simulink model "Sim_AdaptiveFinalazo_ultimo_adaptativo"  (Simulink 7.9)
settings: Solver=ode45  SolverMode=SingleTasking  StartTime=0.0  StopTime=10.0  RelTol=1e-3
values from neighbouring files (symbols this model uses):
  B = [0;1]    [leyDeControl.m]
  gamma = 0.01 *eye(2)    [leyDeControl.m]
  In = 0.002381    [parametros_ultimo.m]
  Kd = 10000    [leyDeControl.m]    (also in parametros_ultimo.m)
  Kn = 0.0347    [parametros_ultimo.m]
  Kp = 100000    [leyDeControl.m]    (also in parametros_ultimo.m)
  Ln = 0.2175    [parametros_ultimo.m]
  Mn = 0.1047708    [parametros_ultimo.m]
  P = lyap(A,Q)    [leyDeControl.m]    (also in parametros_ultimo.m = lyap(a,0.2*eye(2)))
undefined symbols (not defined in the file or in its folder): Kfn
libraries: simulink x4
settings Model: Creator=Harryth  LastModifiedBy=i95sa
settings DataIOCC: SignalLoggingSaveFormat=Dataset
settings OptimizationCC: BlockReduction=off  BooleanDataType=off  ExpressionDepthLimit=128
settings DebuggingCC: SaveWithParameterizedLinksMsg=none  SignalResolutionControl=TryResolveAllWithWarning  SolverPrmCheckMsg=none  FrameProcessingCompatibilityMsg=error  StateNameClashWarn=none
settings HardwareCC: TargetUnknown=on
settings CodeAppCC: CustomSymbolStrType=$N$R$M_T
settings GRTTargetCC: CodeReplacementLibrary=C89/C90 (ANSI)

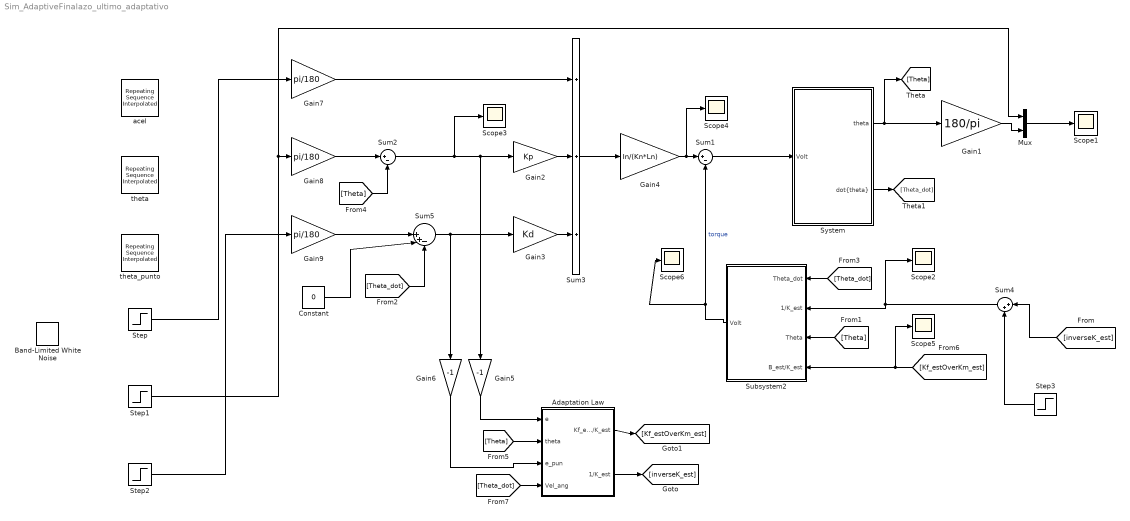
== system Sim_AdaptiveFinalazo_ultimo_adaptativo ==
  Adaptation Law : Subsystem
  Band-Limited White Noise : simulink/Sources/Band-Limited White Noise  Cov=[0.00001]  Ts=0.1  seed=[23341]
  Constant : Constant  Value=0
  Gain1 : Gain  Gain=180/pi
  Gain2 : Gain  Gain=Kp
  Gain3 : Gain  Gain=Kd
  Gain4 : Gain  Gain=In/(Kn*Ln)
  Gain5 : Gain  Gain=-1
  Gain6 : Gain  Gain=-1
  Gain7 : Gain  Gain=pi/180
  Gain8 : Gain  Gain=pi/180
  Gain9 : Gain  Gain=pi/180
  Mux : Mux  Inputs=2
  Scope{1..6} (6 alike) : Scope
      Scope1 settings: TimeRange=auto  MaxDataPoints=5000  SaveName=x1  YMin=-41.89754  YMax=4.65528  SampleTime=-1  DataFormat=Array
      Scope2 settings: TimeRange=auto  MaxDataPoints=5000  SaveName=x  YMin=35.99194  YMax=36.21018  SampleTime=-1  DataFormat=Array
      Scope3 settings: TimeRange=auto  LimitDataPoints=on  MaxDataPoints=5000  SaveToWorkspace=off  SaveName=ScopeData  YMin=-10  YMax=10  SampleTime=-1  DataFormat=Array
      Scope4 settings: TimeRange=auto  LimitDataPoints=on  MaxDataPoints=5000  SaveToWorkspace=off  SaveName=ScopeData  YMin=-4609.88714  YMax=40404.40736  SampleTime=-1  DataFormat=Array
      Scope5 settings: TimeRange=auto  MaxDataPoints=5000  SaveName=x2  YMin=-0.88055  YMax=0.67421  SampleTime=-1  DataFormat=Array
      Scope6 settings: TimeRange=auto  LimitDataPoints=on  MaxDataPoints=5000  SaveToWorkspace=off  SaveName=ScopeData  YMin=-6.67771  YMax=27.31814  SampleTime=-1  DataFormat=Array
  Step : Step  Time=0  After=0  SampleTime=0
  Step1 : Step  Time=0  After=0  SampleTime=0
  Step2 : Step  Time=0  After=0  SampleTime=0
  Step3 : Step  Time=5  After=pi/18  SampleTime=0
  Subsystem2 : Subsystem
  Sum1 : Sum  Inputs=|+-
  Sum2 : Sum  Inputs=|+-
  Sum3 : Sum  Inputs=+++
  Sum4 : Sum  Inputs=|++
  Sum5 : Sum  Inputs=||++-
  System : Subsystem
  acel : simulink/Sources/Repeating Sequence Interpolated  OutValues=|  TimeValues=|  LookUpMeth=Interpolation-Use End Values  tsamp=0.01  OutMin=[]  OutMax=[]  OutDataTypeStr=double  OutputDataTypeScalingMode=double  OutDataType=fixdt(0,8)  OutScaling=2^-10
      OutValues=|
      | [3.12
      | 3.06
      | 3.00
      | 2.93
      | 2.87
      | 2.81
      | 2.75
      | 2.68
      | 2.62
      | 2.56
      | 2.50
      | 2.43
      | 2.37
      | 2.31
      | 2.25
      | 2.18
      | 2.12
      | 2.06
      | 2.00
      | 1.93
      | 1.87
      | 1.81
      | 1.75
      | 1.68
      | 1.62
      | 1.56
      | 1.50
      | 1.44
      | 1.37
      | 1.31
      | 1.25
      | 1.19
      | 1.12
      | 1.06
      | 1.00
      | 0.94
      | 0.87
      | 0.81
      | 0.75
      | 0.69
      | 0.62
      | 0.56
      | 0.50
      | 0.44
      | 0.37
      | 0.31
      | 0.25
      | 0.19
      | 0.12
      | 0.06
      | 0.00
      | -0.06
      | -0.12
      | -0.19
      | -0.25
      | -0.31
      | -0.37
      | -0.44
      | -0.50
      | -0.56
      | -0.62
      | -0.69
      | -0.75
      | -0.81
      | -0.87
      | -0.94
      | -1.00
      | -1.06
      | -1.12
      | -1.19
      | -1.25
      | -1.31
      | -1.37
      | -1.44
      | -1.50
      | -1.56
      | -1.62
      | -1.68
      | -1.75
      | -1.81
      | -1.87
      | -1.93
      | -2.00
      | -2.06
      | -2.12
      | -2.18
      | -2.25
      | -2.31
      | -2.37
      | -2.43
      | -2.50
      | -2.56
      | -2.62
      | -2.68
      | -2.75
      | -2.81
      | -2.87
      | -2.93
      | -3.00
      | -3.06
      | -3.12
      | ].'
      TimeValues=|
      | [0.00
      | 0.10
      | 0.20
      | 0.30
      | 0.40
      | 0.50
      | 0.60
      | 0.70
      | 0.80
      | 0.90
      | 1.00
      | 1.10
      | 1.20
      | 1.30
      | 1.40
      | 1.50
      | 1.60
      | 1.70
      | 1.80
      | 1.90
      | 2.00
      | 2.10
      | 2.20
      | 2.30
      | 2.40
      | 2.50
      | 2.60
      | 2.70
      | 2.80
      | 2.90
      | 3.00
      | 3.10
      | 3.20
      | 3.30
      | 3.40
      | 3.50
      | 3.60
      | 3.70
      | 3.80
      | 3.90
      | 4.00
      | 4.10
      | 4.20
      | 4.30
      | 4.40
      | 4.50
      | 4.60
      | 4.70
      | 4.80
      | 4.90
      | 5.00
      | 5.10
      | 5.20
      | 5.30
      | 5.40
      | 5.50
      | 5.60
      | 5.70
      | 5.80
      | 5.90
      | 6.00
      | 6.10
      | 6.20
      | 6.30
      | 6.40
      | 6.50
      | 6.60
      | 6.70
      | 6.80
      | 6.90
      | 7.00
      | 7.10
      | 7.20
      | 7.30
      | 7.40
      | 7.50
      | 7.60
      | 7.70
      | 7.80
      | 7.90
      | 8.00
      | 8.10
      | 8.20
      | 8.30
      | 8.40
      | 8.50
      | 8.60
      | 8.70
      | 8.80
      | 8.90
      | 9.00
      | 9.10
      | 9.20
      | 9.30
      | 9.40
      | 9.50
      | 9.60
      | 9.70
      | 9.80
      | 9.90
      | 10.00].'
  theta : simulink/Sources/Repeating Sequence Interpolated  OutValues=|  TimeValues=|  LookUpMeth=Interpolation-Use End Values  tsamp=0.01  OutMin=[]  OutMax=[]  OutDataTypeStr=double  OutputDataTypeScalingMode=double  OutDataType=fixdt(0,8)  OutScaling=2^-10
      OutValues=|
      | [-37.00
      | -36.98
      | -36.94
      | -36.86
      | -36.76
      | -36.62
      | -36.46
      | -36.27
      | -36.05
      | -35.81
      | -35.54
      | -35.25
      | -34.93
      | -34.59
      | -34.23
      | -33.84
      | -33.43
      | -33.00
      | -32.55
      | -32.08
      | -31.59
      | -31.08
      | -30.56
      | -30.01
      | -29.45
      | -28.88
      | -28.28
      | -27.67
      | -27.05
      | -26.42
      | -25.77
      | -25.11
      | -24.43
      | -23.75
      | -23.05
      | -22.35
      | -21.63
      | -20.91
      | -20.18
      | -19.44
      | -18.70
      | -17.94
      | -17.19
      | -16.42
      | -15.66
      | -14.89
      | -14.11
      | -13.34
      | -12.56
      | -11.78
      | -11.00
      | -10.22
      | -9.44
      | -8.66
      | -7.89
      | -7.11
      | -6.34
      | -5.58
      | -4.81
      | -4.06
      | -3.30
      | -2.56
      | -1.82
      | -1.09
      | -0.37
      | 0.35
      | 1.05
      | 1.75
      | 2.43
      | 3.11
      | 3.77
      | 4.42
      | 5.05
      | 5.67
      | 6.28
      | 6.88
      | 7.45
      | 8.01
      | 8.56
      | 9.08
      | 9.59
      | 10.08
      | 10.55
      | 11.00
      | 11.43
      | 11.84
      | 12.23
      | 12.59
      | 12.93
      | 13.25
      | 13.54
      | 13.81
      | 14.05
      | 14.27
      | 14.46
      | 14.62
      | 14.76
      | 14.86
      | 14.94
      | 14.98
      | 15.00
      | ].'
      TimeValues=|
      | [0.00
      | 0.10
      | 0.20
      | 0.30
      | 0.40
      | 0.50
      | 0.60
      | 0.70
      | 0.80
      | 0.90
      | 1.00
      | 1.10
      | 1.20
      | 1.30
      | 1.40
      | 1.50
      | 1.60
      | 1.70
      | 1.80
      | 1.90
      | 2.00
      | 2.10
      | 2.20
      | 2.30
      | 2.40
      | 2.50
      | 2.60
      | 2.70
      | 2.80
      | 2.90
      | 3.00
      | 3.10
      | 3.20
      | 3.30
      | 3.40
      | 3.50
      | 3.60
      | 3.70
      | 3.80
      | 3.90
      | 4.00
      | 4.10
      | 4.20
      | 4.30
      | 4.40
      | 4.50
      | 4.60
      | 4.70
      | 4.80
      | 4.90
      | 5.00
      | 5.10
      | 5.20
      | 5.30
      | 5.40
      | 5.50
      | 5.60
      | 5.70
      | 5.80
      | 5.90
      | 6.00
      | 6.10
      | 6.20
      | 6.30
      | 6.40
      | 6.50
      | 6.60
      | 6.70
      | 6.80
      | 6.90
      | 7.00
      | 7.10
      | 7.20
      | 7.30
      | 7.40
      | 7.50
      | 7.60
      | 7.70
      | 7.80
      | 7.90
      | 8.00
      | 8.10
      | 8.20
      | 8.30
      | 8.40
      | 8.50
      | 8.60
      | 8.70
      | 8.80
      | 8.90
      | 9.00
      | 9.10
      | 9.20
      | 9.30
      | 9.40
      | 9.50
      | 9.60
      | 9.70
      | 9.80
      | 9.90
      | 10.00].'
  theta_punto : simulink/Sources/Repeating Sequence Interpolated  OutValues=|  TimeValues=|  LookUpMeth=Interpolation-Use End Values  tsamp=0.01  OutMin=[]  OutMax=[]  OutDataTypeStr=double  OutputDataTypeScalingMode=double  OutDataType=fixdt(0,8)  OutScaling=2^-10
      OutValues=|
      | [0.00
      | 0.31
      | 0.61
      | 0.91
      | 1.20
      | 1.48
      | 1.76
      | 2.03
      | 2.30
      | 2.56
      | 2.81
      | 3.05
      | 3.29
      | 3.53
      | 3.76
      | 3.98
      | 4.19
      | 4.40
      | 4.61
      | 4.80
      | 4.99
      | 5.18
      | 5.35
      | 5.53
      | 5.69
      | 5.85
      | 6.00
      | 6.15
      | 6.29
      | 6.42
      | 6.55
      | 6.67
      | 6.79
      | 6.90
      | 7.00
      | 7.10
      | 7.19
      | 7.27
      | 7.35
      | 7.42
      | 7.49
      | 7.55
      | 7.60
      | 7.65
      | 7.69
      | 7.72
      | 7.75
      | 7.77
      | 7.79
      | 7.80
      | 7.80
      | 7.80
      | 7.79
      | 7.77
      | 7.75
      | 7.72
      | 7.69
      | 7.65
      | 7.60
      | 7.55
      | 7.49
      | 7.42
      | 7.35
      | 7.27
      | 7.19
      | 7.10
      | 7.00
      | 6.90
      | 6.79
      | 6.67
      | 6.55
      | 6.42
      | 6.29
      | 6.15
      | 6.00
      | 5.85
      | 5.69
      | 5.53
      | 5.35
      | 5.18
      | 4.99
      | 4.80
      | 4.61
      | 4.40
      | 4.19
      | 3.98
      | 3.76
      | 3.53
      | 3.29
      | 3.05
      | 2.81
      | 2.56
      | 2.30
      | 2.03
      | 1.76
      | 1.48
      | 1.20
      | 0.91
      | 0.61
      | 0.31
      | 0.00
      | ].'
      TimeValues=|
      | [0.00
      | 0.10
      | 0.20
      | 0.30
      | 0.40
      | 0.50
      | 0.60
      | 0.70
      | 0.80
      | 0.90
      | 1.00
      | 1.10
      | 1.20
      | 1.30
      | 1.40
      | 1.50
      | 1.60
      | 1.70
      | 1.80
      | 1.90
      | 2.00
      | 2.10
      | 2.20
      | 2.30
      | 2.40
      | 2.50
      | 2.60
      | 2.70
      | 2.80
      | 2.90
      | 3.00
      | 3.10
      | 3.20
      | 3.30
      | 3.40
      | 3.50
      | 3.60
      | 3.70
      | 3.80
      | 3.90
      | 4.00
      | 4.10
      | 4.20
      | 4.30
      | 4.40
      | 4.50
      | 4.60
      | 4.70
      | 4.80
      | 4.90
      | 5.00
      | 5.10
      | 5.20
      | 5.30
      | 5.40
      | 5.50
      | 5.60
      | 5.70
      | 5.80
      | 5.90
      | 6.00
      | 6.10
      | 6.20
      | 6.30
      | 6.40
      | 6.50
      | 6.60
      | 6.70
      | 6.80
      | 6.90
      | 7.00
      | 7.10
      | 7.20
      | 7.30
      | 7.40
      | 7.50
      | 7.60
      | 7.70
      | 7.80
      | 7.90
      | 8.00
      | 8.10
      | 8.20
      | 8.30
      | 8.40
      | 8.50
      | 8.60
      | 8.70
      | 8.80
      | 8.90
      | 9.00
      | 9.10
      | 9.20
      | 9.30
      | 9.40
      | 9.50
      | 9.60
      | 9.70
      | 9.80
      | 9.90
      | 10.00].'
  wires:
  System/2("dot{theta}") -> [Theta_dot]
  Sum1/1 -> System/1(Volt)
  Subsystem2/1(Volt) -> Scope6/1, Sum1/2  "torque"
  Sum3/1 -> Gain4/1
  Step/1 -> Gain7/1
  Sum4/1 -> Scope2/1, Subsystem2/2(1/K_est)
  [Theta] -> Subsystem2/3(Theta)
  [Theta_dot] -> Subsystem2/1(Theta_dot)
  [Kf_estOverKm_est] -> Scope5/1, Subsystem2/4(B_est/K_est)
  System/1(theta) -> Gain1/1, [Theta]
  [Theta] -> Sum2/2
  [Theta_dot] -> Sum5/3
  Gain2/1 -> Sum3/2
  Gain3/1 -> Sum3/3
  Gain4/1 -> Scope4/1, Sum1/1
  Step1/1 -> Mux/1, Gain8/1
  Step2/1 -> Gain9/1
  Sum5/1 -> Gain3/1, Gain6/1
  [Theta] -> Adaptation Law/2(theta)
  Sum2/1 -> Gain2/1, Gain5/1, Scope3/1
  [Theta_dot] -> Adaptation Law/4("Vel_ang ")
  Gain5/1 -> Adaptation Law/1(e)
  Gain6/1 -> Adaptation Law/3("e_pun ")
  Adaptation Law/1(Kf_est/K_est) -> [Kf_estOverKm_est]
  Adaptation Law/2(1/K_est) -> [inverseK_est]
  Gain7/1 -> Sum3/1
  Gain8/1 -> Sum2/1
  Gain9/1 -> Sum5/1
  Mux/1 -> Scope1/1
  Gain1/1 -> Mux/2
  Constant/1 -> Sum5/2
  [inverseK_est] -> Sum4/1
  Step3/1 -> Sum4/2

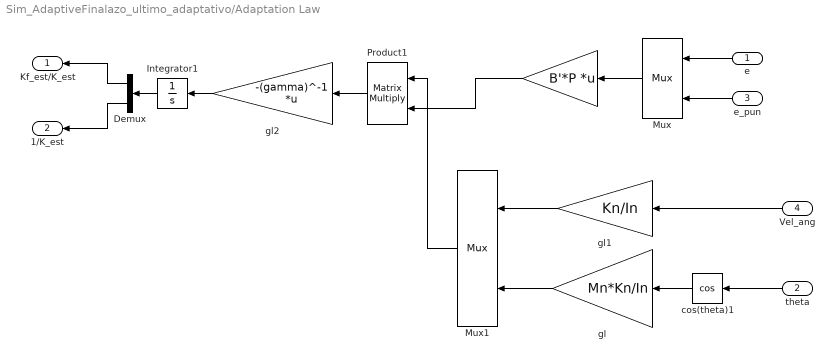
== system Sim_AdaptiveFinalazo_ultimo_adaptativo/Adaptation Law ==
  e : Inport
  theta : Inport  Port=2
  "e_pun " : Inport  Port=3
  "Vel_ang " : Inport  Port=4
  " " : Gain  Gain=B'*P  Multiplication=Matrix(K*u)
  Demux : Demux  Outputs=2
  Integrator1 : Integrator  InitialCondition=[Kfn/Kn ; 1/Kn]
  Mux : Mux  Inputs=2
      settings: DisplayOption=signals
  Mux1 : Mux  Inputs=2
      settings: DisplayOption=signals
  Product1 : Product  Multiplication=Matrix(*)  RndMeth=Zero
  cos(theta)1 : Trigonometry  Operator=cos
  gl : Gain  Gain=Mn*Kn/In
  gl1 : Gain  Gain=Kn/In
  gl2 : Gain  Gain=-(gamma)^-1  Multiplication=Matrix(K*u)
  Kf_est/K_est : Outport
  1/K_est : Outport  Port=2
  wires:
  cos(theta)1/1 -> gl/1
  theta/1 -> cos(theta)1/1
  "Vel_ang "/1 -> gl1/1
  e/1 -> Mux/1
  "e_pun "/1 -> Mux/2
  Mux/1 -> " "/1
  gl1/1 -> Mux1/1
  gl/1 -> Mux1/2
  Integrator1/1 -> Demux/1
  Demux/1 -> Kf_est/K_est/1
  Demux/2 -> 1/K_est/1
  gl2/1 -> Integrator1/1
  Mux1/1 -> Product1/1
  " "/1 -> Product1/2
  Product1/1 -> gl2/1

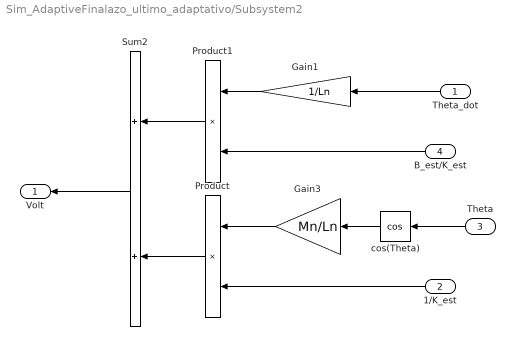
== system Sim_AdaptiveFinalazo_ultimo_adaptativo/Subsystem2 ==
  Theta_dot : Inport
  1/K_est : Inport  Port=2
  Theta : Inport  Port=3
  B_est/K_est : Inport  Port=4
  Gain1 : Gain  Gain=1/Ln
  Gain3 : Gain  Gain=Mn/Ln
  Product : Product  RndMeth=Zero
  Product1 : Product  RndMeth=Zero
  Sum2 : Sum
  cos(Theta) : Trigonometry  Operator=cos
  Volt : Outport
  wires:
  cos(Theta)/1 -> Gain3/1
  Gain3/1 -> Product/1
  Product/1 -> Sum2/2
  Theta_dot/1 -> Gain1/1
  Theta/1 -> cos(Theta)/1
  Sum2/1 -> Volt/1
  1/K_est/1 -> Product/2
  Gain1/1 -> Product1/1
  Product1/1 -> Sum2/1
  B_est/K_est/1 -> Product1/2

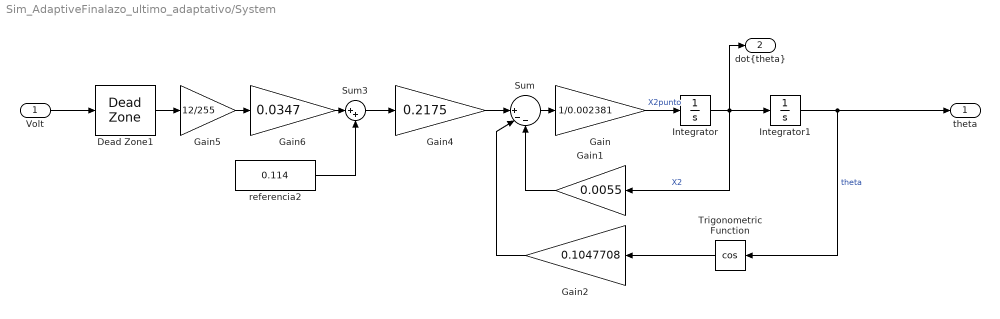
== system Sim_AdaptiveFinalazo_ultimo_adaptativo/System ==
  Volt : Inport
  Dead Zone1 : DeadZone  LowerValue=0  UpperValue=0  SaturateOnIntegerOverflow=on
  Gain : Gain  Gain=1/0.002381
  Gain1 : Gain  Gain=0.0055
  Gain2 : Gain  Gain=0.1047708
  Gain4 : Gain  Gain=0.2175
  Gain5 : Gain  Gain=12/255
  Gain6 : Gain  Gain=0.0347
  Integrator : Integrator
  Integrator1 : Integrator  InitialCondition=-0.65
  Sum : Sum  Inputs=||+--
  Sum3 : Sum  Inputs=|++
  Trigonometric Function : Trigonometry  Operator=cos
  referencia2 : Constant  Value=0.114
  theta : Outport
  "dot{theta}" : Outport  Port=2
  wires:
  Sum/1 -> Gain/1
  Gain/1 -> Integrator/1  "X2punto"
  Integrator/1 -> "dot{theta}"/1, Integrator1/1, Gain1/1  "X2"
  Trigonometric Function/1 -> Gain2/1
  Gain1/1 -> Sum/3
  Integrator1/1 -> Trigonometric Function/1, theta/1  "theta"
  Gain2/1 -> Sum/2
  Gain4/1 -> Sum/1
  referencia2/1 -> Sum3/2
  Sum3/1 -> Gain4/1
  Gain5/1 -> Gain6/1
  Gain6/1 -> Sum3/1
  Dead Zone1/1 -> Gain5/1
  Volt/1 -> Dead Zone1/1
